simulink model "GSPI"  (R2015b)
settings: Solver=ode4  StartTime=0.0  StopTime=TMax  FixedStep=DT  MaxStep=DT  RelTol=1e-3
values from neighbouring files (symbols this model uses):
  DT = fscanf(fid,'    [YY_Read_FAST_Input.m]
  NDOF = 24    [YY_Read_FAST_Input.m]
  NumOuts = 2    [Reduced4to3_2DOF_18.mat]    (also in YY_Read_FAST_Input.m = 1)
  OutList = {}    [YY_Read_FAST_Input.m]
  q_init = zeros(1,NDOF)    [YY_Read_FAST_Input.m]
  qdot_init = zeros(1,NDOF)    [YY_Read_FAST_Input.m]
undefined symbols (not defined in the file or in its folder): strmatch
settings Model: Creator=elemist  LastModifiedBy=yuy13010
settings DataIOCC: SaveFormat=Array  SignalLoggingSaveFormat=ModelDataLogs  SaveOutput=off  SaveTime=off  SignalLoggingName=sigsOut
settings OptimizationCC: ExpressionDepthLimit=2147483647
settings DebuggingCC: SaveWithParameterizedLinksMsg=none  UnderspecifiedInitializationDetection=Classic  MergeDetectMultiDrivingBlocksExec=none  SignalResolutionControl=TryResolveAllWithWarning  MultiTaskDSMMsg=warning  MultiTaskCondExecSysMsg=none  FcnCallInpInsideContextMsg=UseLocalSettings  StateNameClashWarn=warning
settings HardwareCC: ProdBitPerPointer=32  ProdLargestAtomicFloat=None  ProdIntDivRoundTo=Undefined  ProdEndianess=Unspecified  ProdWordSize=32  ProdHWDeviceType=32-bit Generic  TargetUnknown=on
settings GRTTargetCC: GeneratePreprocessorConditionals=Disable all  CombineOutputUpdateFcns=off  GRTInterface=on
settings ConfigComp: CovModelRefEnable=Off

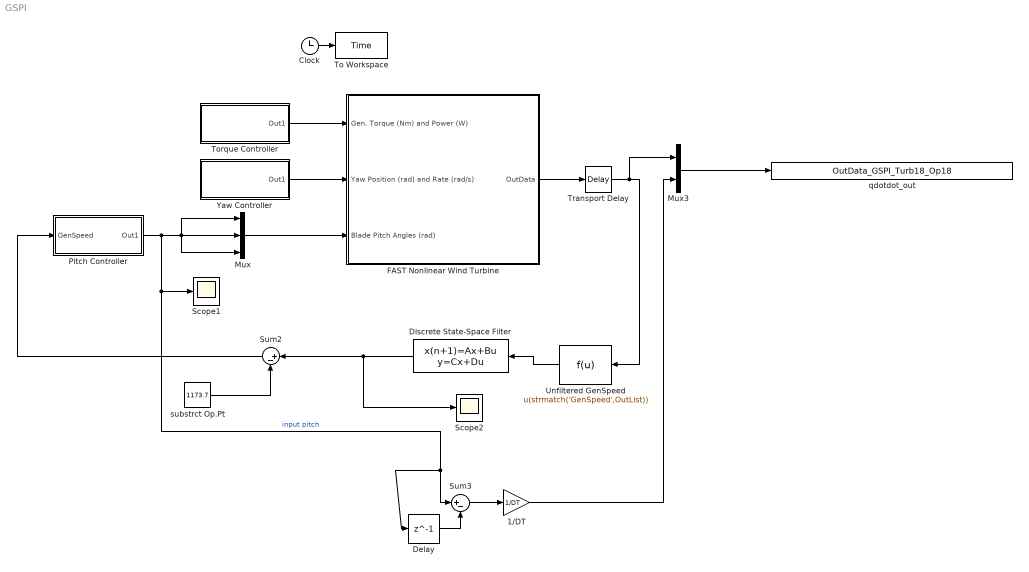
== system GSPI ==
  1/DT : Gain  Gain=1/DT  SaturateOnIntegerOverflow=on  OutDataTypeStr=Inherit: Same as input  ParamDataTypeStr=Inherit: Same as input
  Clock : Clock
  Delay : Delay  DelayLength=1
  Discrete State-Space Filter : DiscreteStateSpace  A=0.9806  B=0.0194  C=0.9806  D=0.0194  SampleTime=DT
  FAST Nonlinear Wind Turbine : Subsystem
  Mux : Mux  Inputs=3
  Mux3 : Mux  Inputs=2
  Pitch Controller : Subsystem  TreatAsAtomicUnit=on
  Scope1 : Scope
  Scope2 : Scope
  Sum2 : Sum  Inputs=|+-  SampleTime=DT
  Sum3 : Sum  Inputs=|+-  SampleTime=DT
  To Workspace : ToWorkspace  VariableName=Time  SampleTime=-1
  Torque Controller : Subsystem
  Transport Delay : TransportDelay  DelayTime=0.02
  Unfiltered GenSpeed : Fcn  Expr=u(strmatch('GenSpeed',OutList))  SampleTime=DT
  Yaw Controller : Subsystem
  qdotdot_out : ToWorkspace  VariableName=OutData_GSPI_Turb18_Op18  SampleTime=-1
  substrct Op.Pt : Constant  Value=1173.7
  wires:
  Clock/1 -> To Workspace/1
  Torque Controller/1(Out1) -> FAST Nonlinear Wind Turbine/1(Gen. Torque (Nm) and Power (W))
  Yaw Controller/1(Out1) -> FAST Nonlinear Wind Turbine/2(Yaw Position (rad) and Rate (rad/s))
  Mux/1 -> FAST Nonlinear Wind Turbine/3(Blade Pitch Angles (rad))
  FAST Nonlinear Wind Turbine/1(OutData) -> Transport Delay/1
  substrct Op.Pt/1 -> Sum2/2
  Unfiltered GenSpeed/1 -> Discrete State-Space Filter/1
  Sum2/1 -> Pitch Controller/1(GenSpeed)
  Discrete State-Space Filter/1 -> Scope2/1, Sum2/1
  Pitch Controller/1(Out1) -> Delay/1, Sum3/1, Scope1/1, Mux/1, Mux/3, Mux/2  "input pitch"
  Delay/1 -> Sum3/2
  Sum3/1 -> 1/DT/1
  1/DT/1 -> Mux3/2
  Mux3/1 -> qdotdot_out/1
  Transport Delay/1 -> Mux3/1, Unfiltered GenSpeed/1

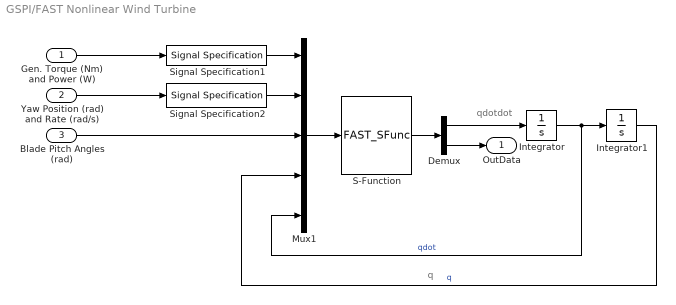
== system GSPI/FAST Nonlinear Wind Turbine ==
  note: qdotdot
  note: q
  Gen. Torque (Nm) and Power (W) : Inport
  Yaw Position (rad) and Rate (rad/s) : Inport  Port=2
  Blade Pitch Angles (rad) : Inport  Port=3
  Demux : Demux  Outputs=[NDOF, NumOuts]
  Integrator : Integrator  InitialCondition=qdot_init
  Integrator1 : Integrator  InitialCondition=q_init
  Mux1 : Mux  Inputs=5
  S-Function : S-Function  FunctionName=FAST_SFunc  SFunctionDeploymentMode=off  EnableBusSupport=off
  Signal Specification1 : SignalSpecification  OutDataTypeStr=double  Dimensions=2
  Signal Specification2 : SignalSpecification  OutDataTypeStr=double  Dimensions=2
  OutData : Outport
  wires:
  Integrator/1 -> Integrator1/1, Mux1/5  "qdot"
  Gen. Torque (Nm) and Power (W)/1 -> Signal Specification1/1
  S-Function/1 -> Demux/1
  Demux/1 -> Integrator/1
  Demux/2 -> OutData/1
  Mux1/1 -> S-Function/1
  Blade Pitch Angles (rad)/1 -> Mux1/3
  Yaw Position (rad) and Rate (rad/s)/1 -> Signal Specification2/1
  Integrator1/1 -> Mux1/4  "q"
  Signal Specification1/1 -> Mux1/1
  Signal Specification2/1 -> Mux1/2

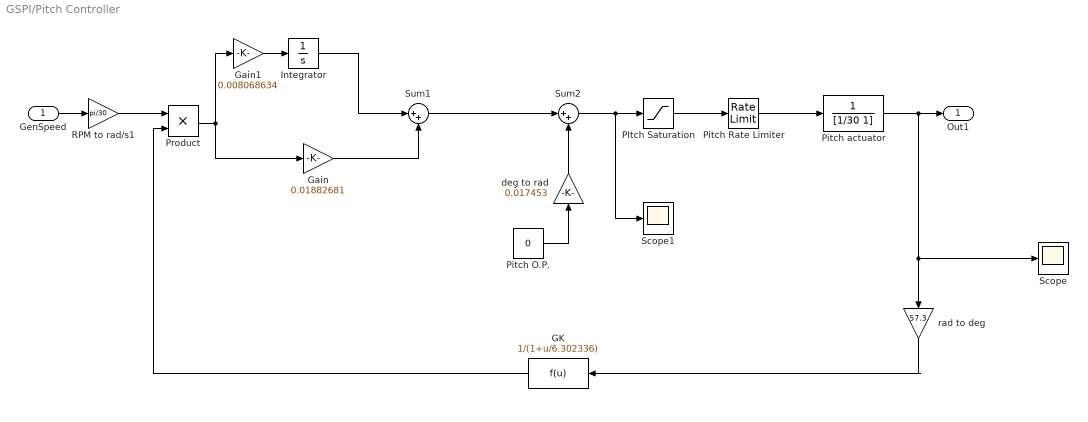
== system GSPI/Pitch Controller ==
  GenSpeed : Inport
  GK : Fcn  Expr=1/(1+u/6.302336)  SampleTime=DT
  Gain : Gain  Gain=0.01882681  SampleTime=DT
  Gain1 : Gain  Gain=0.008068634
  Integrator : Integrator
  PItch Saturation : Saturate  UpperLimit=1.570796  LowerLimit=0  SampleTime=DT
  Pitch O.P. : Constant  Value=0
  Pitch Rate Limiter : RateLimiter  RisingSlewLimit=0.1396263  FallingSlewLimit=-0.1396263  SampleTimeMode=inherited
  Pitch actuator : TransferFcn  Denominator=[1/30 1]
  Product : Product
  RPM to rad/s1 : Gain  Gain=pi/30  SaturateOnIntegerOverflow=on  OutDataTypeStr=Inherit: Same as input  ParamDataTypeStr=Inherit: Same as input
  Scope : Scope
  Scope1 : Scope
  Sum1 : Sum  Inputs=|++
  Sum2 : Sum  Inputs=|++
  deg to rad : Gain  Gain=0.017453  SaturateOnIntegerOverflow=on  OutDataTypeStr=Inherit: Same as input  ParamDataTypeStr=Inherit: Same as input
  "rad to deg " : Gain  Gain=57.3  SaturateOnIntegerOverflow=on  OutDataTypeStr=Inherit: Same as input  ParamDataTypeStr=Inherit: Same as input
  Out1 : Outport
  wires:
  GenSpeed/1 -> RPM to rad/s1/1
  Gain1/1 -> Integrator/1
  Integrator/1 -> Sum1/1
  Gain/1 -> Sum1/2
  PItch Saturation/1 -> Pitch Rate Limiter/1
  Sum2/1 -> Scope1/1, PItch Saturation/1
  Sum1/1 -> Sum2/1
  Pitch O.P./1 -> deg to rad/1
  Pitch Rate Limiter/1 -> Pitch actuator/1
  Pitch actuator/1 -> Out1/1, "rad to deg "/1, Scope/1
  GK/1 -> Product/2
  RPM to rad/s1/1 -> Product/1
  Product/1 -> Gain1/1, Gain/1
  deg to rad/1 -> Sum2/2
  "rad to deg "/1 -> GK/1

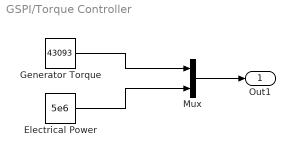
== system GSPI/Torque Controller ==
  Electrical Power : Constant  Value=5e6
  Generator Torque : Constant  Value=43093
  Mux : Mux  Inputs=2
  Out1 : Outport
  wires:
  Mux/1 -> Out1/1
  Generator Torque/1 -> Mux/1
  Electrical Power/1 -> Mux/2

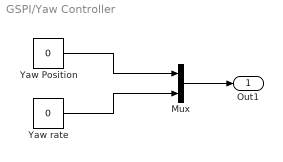
== system GSPI/Yaw Controller ==
  Mux : Mux  Inputs=2
  Yaw Position : Constant  Value=0
  Yaw rate : Constant  Value=0
  Out1 : Outport
  wires:
  Mux/1 -> Out1/1
  Yaw Position/1 -> Mux/1
  Yaw rate/1 -> Mux/2
